simulink model "UAV_Autopilot"  (R2025a)
settings: Solver=ode4  StartTime=0.0  StopTime=120  FixedStep=0.01  RelTol=1e-3
model workspace (MAT data in the model file):
  P.g = 9.81
  P.mass = 13.5
  P.Jx = 0.8244
  P.Jy = 1.135
  P.Jz = 1.759
  P.Jxz = 0.1204
  P.S_wing = 0.55
  P.b = 2.8956
  P.c = 0.18994
  P.S_prop = 0.2027
  P.rho = 1.2682
  P.e_oswald = 0.9
  P.AR = 15.2445442909
  P.C_L_0 = 0.28
  P.C_L_alpha = 3.45
  P.C_L_q = 0
  P.C_L_delta_e = -0.36
  P.C_D_0 = 0.03
  P.C_D_alpha = 0.3
  P.C_D_p = 0.0437
  P.C_D_q = 0
  P.C_D_delta_e = 0
  P.C_m_0 = -0.02338
  P.C_m_alpha = -0.38
  P.C_m_q = -3.6
  P.C_m_delta_e = -0.5
  P.C_Y_0 = 0
  P.C_Y_beta = -0.98
  P.C_Y_p = 0
  P.C_Y_r = 0
  P.C_Y_delta_a = 0
  P.C_Y_delta_r = -0.17
  P.C_ell_0 = 0
  P.C_ell_beta = -0.12
  P.C_ell_p = -0.26
  P.C_ell_r = 0.14
  P.C_ell_delta_a = 0.08
  P.C_ell_delta_r = 0.105
  P.C_n_0 = 0
  P.C_n_beta = 0.25
  P.C_n_p = 0.022
  P.C_n_r = -0.35
  P.C_n_delta_a = 0.06
  P.C_n_delta_r = -0.032
  P.C_prop = 1
  P.k_motor = 80
  P.M = 50
  P.epsilon = 0.1592
  P.alpha0 = 0.4712
  P.limits.delta_e = 0.436332312999
  P.limits.delta_a = 0.436332312999
  P.limits.delta_r = 0.436332312999
  P.limits.delta_t_min = 0
  P.limits.delta_t_max = 1
  P.limits.phi_cmd = 0.610865238198
  P.limits.theta_cmd = 0.349065850399
  P.control.manual.roll.Kp = 1.05
  P.control.manual.roll.Ki = 0.12
  P.control.manual.roll.Kd = 0.18
  P.control.manual.pitch.Kp = 1.65
  P.control.manual.pitch.Ki = 0.1
  P.control.manual.pitch.Kd = 0.28
  P.control.manual.course.Kp = 1.2
  P.control.manual.course.Ki = 0.08
  P.control.manual.altitude.Kp = 0.02
  P.control.manual.altitude.Ki = 0.0015
  P.control.manual.airspeed.Kp = 0.07
  P.control.manual.airspeed.Ki = 0.025
  P.control.roll.Kp = 1.05
  P.control.roll.Ki = 0.12
  P.control.roll.Kd = 0.18
  P.control.pitch.Kp = 1.65
  P.control.pitch.Ki = 0.1
  P.control.pitch.Kd = 0.28
  P.control.course.Kp = 1.2
  P.control.course.Ki = 0.08
  P.control.altitude.Kp = 0.02
  P.control.altitude.Ki = 0.0015
  P.control.airspeed.Kp = 0.07
  P.control.airspeed.Ki = 0.025
  P.control.profile = 'manual'
  P.trim.Va = 25
  P.trim.h = 100
  P.trim.alpha = 0.0823209529795
  P.trim.theta = 0.0823209529869
  P.trim.delta_e = -0.10932392429
  P.trim.delta_t = 0.333522593056
  P.trim.x0 = [0; 0; -100; 24.9153385857; 0; 2.05570016348; 0; 0.0823209529869; 0; 0; 0; 0]
  P.trim.residual = 1.21239568629e-09
  P.trim.cost = 4.97403810969e-18
  P.trim.exitflag = 1
  P.sim.dt = 0.01
  P.sim.duration = 120
  P.sim.scenario = 'nominal'
  P.sim.wind_ned = [0; 0; 0]
  P.sim.Va_cmd = 25
  P.sim.h0 = 100
  P.sim.waypoint_radius = 40
  P.sim.waypoints = [400  0  120; 400  400  120; 0  400  140; 0  0  120]
  P.tuning.dt = 0.02
  P.tuning.MaxIterations = 14
  P.tuning.MaxFunctionEvaluations = 24
  P.tuning.TolX = 0.001
  P.tuning.TolFun = 0.001
  P.tuning.lower_multiplier.Kp = 0.25
  P.tuning.lower_multiplier.Ki = 0.1
  P.tuning.lower_multiplier.Kd = 0.25
  P.tuning.upper_multiplier.Kp = 4
  P.tuning.upper_multiplier.Ki = 5
  P.tuning.upper_multiplier.Kd = 4
  wind_ned = [0; 0; 0]
  x0 = [0; 0; -100; 24.9153385857; 0; 2.05570016348; 0; 0.0823209529869; 0; 0; 0; 0]
values from neighbouring files (symbols this model uses):
  P = aircraft_parameters()    [build_model.m]
undefined symbols (not defined in the file or in its folder): air_data, aircraft_dynamics, command_guidance, limit_actuators
settings Model: Creator=Priyanshi Paul  LastModifiedBy=Priyanshi Paul

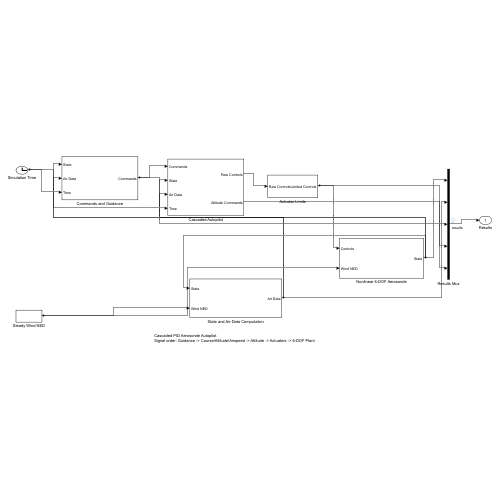
[thumbnail: Simulink's stored preview of the top-level diagram]
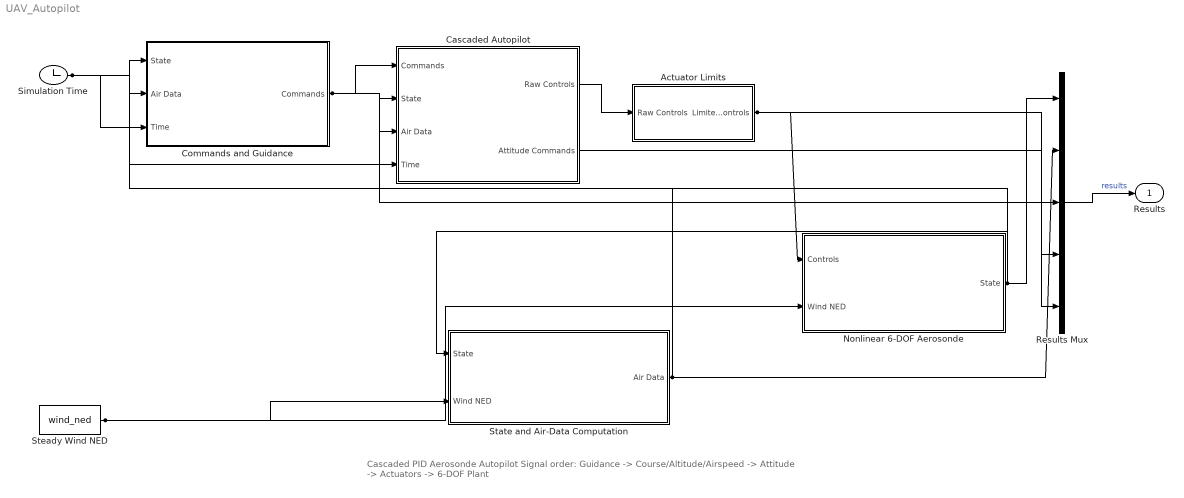
== system UAV_Autopilot ==
  note: Cascaded PID Aerosonde Autopilot
      | Signal order: Guidance -> Course/Altitude/Airspeed -> Attitude -> Actuators -> 6-DOF Plant
  Actuator Limits : Subsystem
  Cascaded Autopilot : Subsystem
  Commands and Guidance : Subsystem
  Nonlinear 6-DOF Aerosonde : Subsystem
  Results Mux : Mux  Inputs=5
  Simulation Time : Clock
  State and Air-Data Computation : Subsystem
  Steady Wind NED : Constant  Value=wind_ned
  Results : Outport
  wires:
  Simulation Time/1 -> Commands and Guidance/3(Time), Cascaded Autopilot/4(Time)
  Steady Wind NED/1 -> Nonlinear 6-DOF Aerosonde/2(Wind NED), State and Air-Data Computation/2(Wind NED)
  Nonlinear 6-DOF Aerosonde/1(State) -> State and Air-Data Computation/1(State), Commands and Guidance/1(State), Cascaded Autopilot/2(State), Results Mux/1
  State and Air-Data Computation/1(Air Data) -> Commands and Guidance/2(Air Data), Cascaded Autopilot/3(Air Data), Results Mux/2
  Commands and Guidance/1(Commands) -> Cascaded Autopilot/1(Commands), Results Mux/3
  Cascaded Autopilot/1(Raw Controls) -> Actuator Limits/1(Raw Controls)
  Cascaded Autopilot/2(Attitude Commands) -> Results Mux/4
  Actuator Limits/1(Limited Controls) -> Nonlinear 6-DOF Aerosonde/1(Controls), Results Mux/5
  Results Mux/1 -> Results/1  "results"

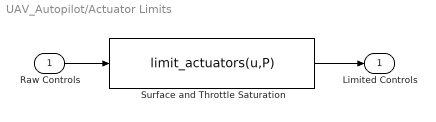
== system UAV_Autopilot/Actuator Limits ==
  Raw Controls : Inport
  Surface and Throttle Saturation : MATLABFcn  MATLABFcn=limit_actuators(u,P)  OutputDimensions=4
  Limited Controls : Outport
  wires:
  Raw Controls/1 -> Surface and Throttle Saturation/1
  Surface and Throttle Saturation/1 -> Limited Controls/1

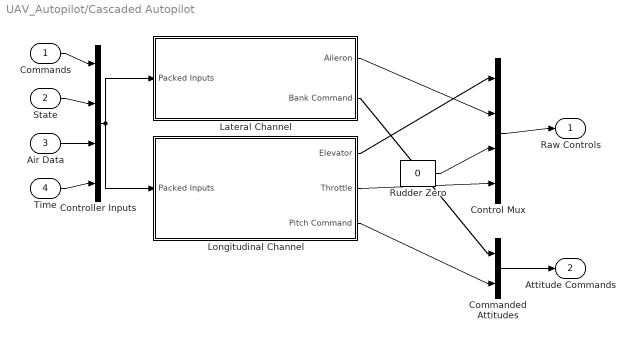
== system UAV_Autopilot/Cascaded Autopilot ==
  Commands : Inport
  State : Inport  Port=2
  Air Data : Inport  Port=3
  Time : Inport  Port=4
  Commanded Attitudes : Mux  Inputs=2
  Control Mux : Mux
  Controller Inputs : Mux
  Lateral Channel : Subsystem
  Longitudinal Channel : Subsystem
  Rudder Zero : Constant  Value=0
  Raw Controls : Outport
  Attitude Commands : Outport  Port=2
  wires:
  Commands/1 -> Controller Inputs/1
  State/1 -> Controller Inputs/2
  Air Data/1 -> Controller Inputs/3
  Time/1 -> Controller Inputs/4
  Controller Inputs/1 -> Lateral Channel/1(Packed Inputs), Longitudinal Channel/1(Packed Inputs)
  Longitudinal Channel/1(Elevator) -> Control Mux/1
  Lateral Channel/1(Aileron) -> Control Mux/2
  Rudder Zero/1 -> Control Mux/3
  Longitudinal Channel/2(Throttle) -> Control Mux/4
  Lateral Channel/2(Bank Command) -> Commanded Attitudes/1
  Longitudinal Channel/3(Pitch Command) -> Commanded Attitudes/2
  Control Mux/1 -> Raw Controls/1
  Commanded Attitudes/1 -> Attitude Commands/1

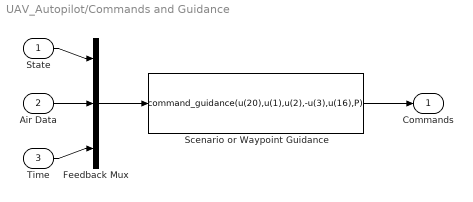
== system UAV_Autopilot/Commands and Guidance ==
  State : Inport
  Air Data : Inport  Port=2
  Time : Inport  Port=3
  Feedback Mux : Mux  Inputs=3
  Scenario or Waypoint Guidance : MATLABFcn  MATLABFcn=command_guidance(u(20),u(1),u(2),-u(3),u(16),P)  OutputDimensions=4
  Commands : Outport
  wires:
  State/1 -> Feedback Mux/1
  Air Data/1 -> Feedback Mux/2
  Time/1 -> Feedback Mux/3
  Feedback Mux/1 -> Scenario or Waypoint Guidance/1
  Scenario or Waypoint Guidance/1 -> Commands/1

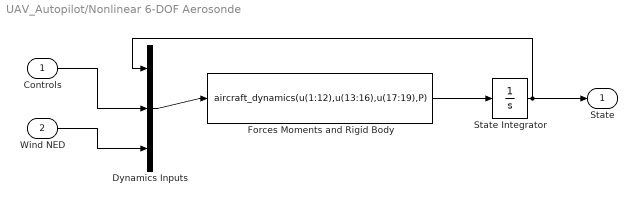
== system UAV_Autopilot/Nonlinear 6-DOF Aerosonde ==
  Controls : Inport
  Wind NED : Inport  Port=2
  Dynamics Inputs : Mux  Inputs=3
  Forces Moments and Rigid Body : MATLABFcn  MATLABFcn=aircraft_dynamics(u(1:12),u(13:16),u(17:19),P)  OutputDimensions=12
  State Integrator : Integrator  InitialCondition=x0
  State : Outport
  wires:
  State Integrator/1 -> Dynamics Inputs/1, State/1
  Controls/1 -> Dynamics Inputs/2
  Wind NED/1 -> Dynamics Inputs/3
  Dynamics Inputs/1 -> Forces Moments and Rigid Body/1
  Forces Moments and Rigid Body/1 -> State Integrator/1

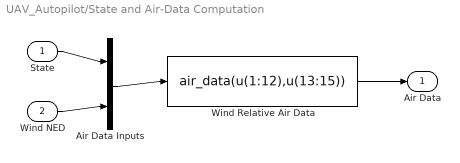
== system UAV_Autopilot/State and Air-Data Computation ==
  State : Inport
  Wind NED : Inport  Port=2
  Air Data Inputs : Mux  Inputs=2
  Wind Relative Air Data : MATLABFcn  MATLABFcn=air_data(u(1:12),u(13:15))  OutputDimensions=7
  Air Data : Outport
  wires:
  State/1 -> Air Data Inputs/1
  Wind NED/1 -> Air Data Inputs/2
  Air Data Inputs/1 -> Wind Relative Air Data/1
  Wind Relative Air Data/1 -> Air Data/1

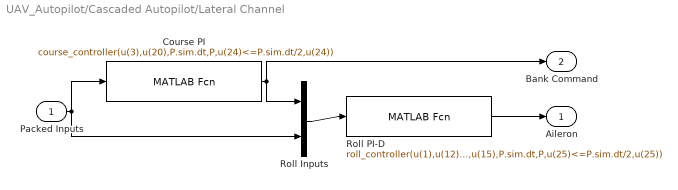
== system UAV_Autopilot/Cascaded Autopilot/Lateral Channel ==
  Packed Inputs : Inport
  Course PI : MATLABFcn  MATLABFcn=course_controller(u(3),u(20),P.sim.dt,P,u(24)<=P.sim.dt/2,u(24))  OutputDimensions=1
  Roll Inputs : Mux  Inputs=2
  Roll PI-D : MATLABFcn  MATLABFcn=roll_controller(u(1),u(12),u(15),P.sim.dt,P,u(25)<=P.sim.dt/2,u(25))  OutputDimensions=1
  Aileron : Outport
  Bank Command : Outport  Port=2
  wires:
  Packed Inputs/1 -> Course PI/1, Roll Inputs/2
  Course PI/1 -> Roll Inputs/1, Bank Command/1
  Roll Inputs/1 -> Roll PI-D/1
  Roll PI-D/1 -> Aileron/1

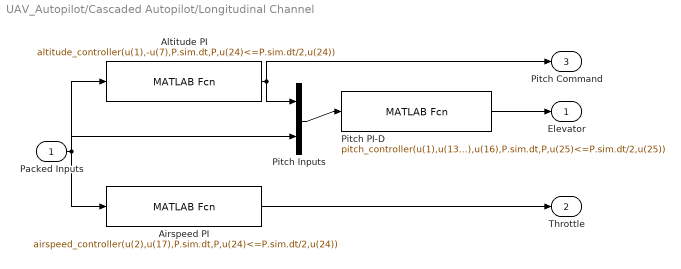
== system UAV_Autopilot/Cascaded Autopilot/Longitudinal Channel ==
  Packed Inputs : Inport
  Airspeed PI : MATLABFcn  MATLABFcn=airspeed_controller(u(2),u(17),P.sim.dt,P,u(24)<=P.sim.dt/2,u(24))  OutputDimensions=1
  Altitude PI : MATLABFcn  MATLABFcn=altitude_controller(u(1),-u(7),P.sim.dt,P,u(24)<=P.sim.dt/2,u(24))  OutputDimensions=1
  Pitch Inputs : Mux  Inputs=2
  Pitch PI-D : MATLABFcn  MATLABFcn=pitch_controller(u(1),u(13),u(16),P.sim.dt,P,u(25)<=P.sim.dt/2,u(25))  OutputDimensions=1
  Elevator : Outport
  Throttle : Outport  Port=2
  Pitch Command : Outport  Port=3
  wires:
  Packed Inputs/1 -> Altitude PI/1, Pitch Inputs/2, Airspeed PI/1
  Altitude PI/1 -> Pitch Inputs/1, Pitch Command/1
  Pitch Inputs/1 -> Pitch PI-D/1
  Pitch PI-D/1 -> Elevator/1
  Airspeed PI/1 -> Throttle/1
